simulink model "lab2_5_observer"  (R2023a)
settings: Solver=VariableStepAuto  StartTime=0.0  StopTime=2  RelTol=1e-3
values from neighbouring files (symbols this model uses):
  A = eye(3) + Ts * A    [part_deriv.m]
undefined symbols (not defined in the file or in its folder): B, C, K, L, u0, x10, x20, x30
settings Model: Creator=bz  LastModifiedBy=bz

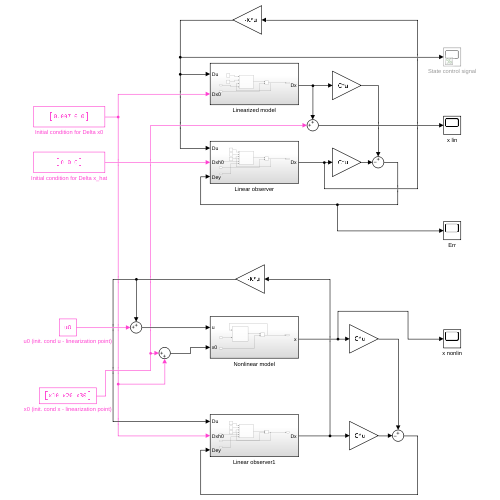
[thumbnail: Simulink's stored preview of the top-level diagram]
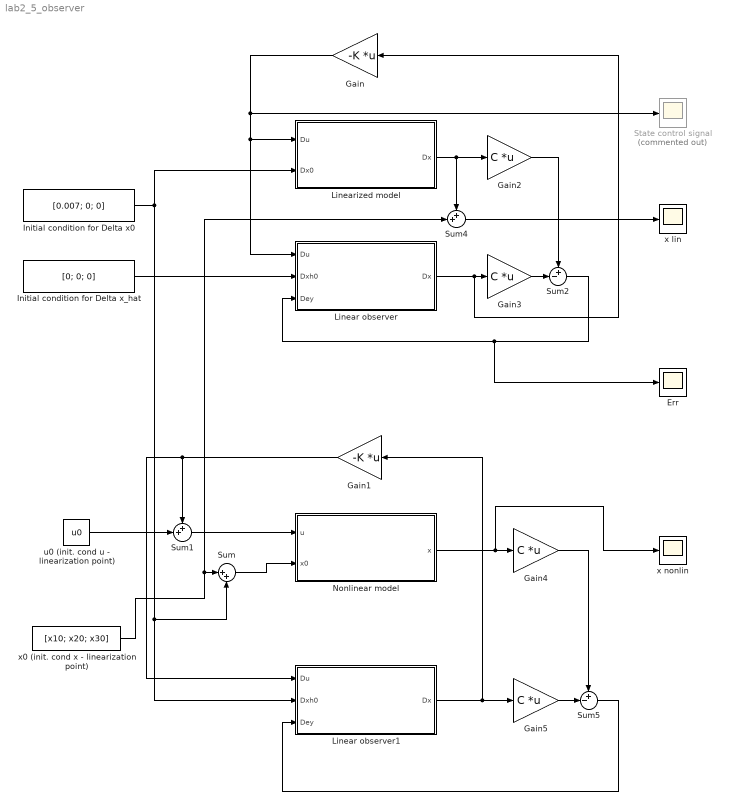
== system lab2_5_observer ==
  Err : Scope
  Gain : Gain  Gain=-K  Multiplication=Matrix(K*u)
  Gain1 : Gain  Gain=-K  Multiplication=Matrix(K*u)
  Gain{2..5} (4 alike) : Gain  Gain=C  Multiplication=Matrix(K*u)
  Initial condition for Delta x0 : Constant  Value=[0.007; 0; 0]
  Initial condition for Delta x_hat : Constant  Value=[0; 0; 0]
  Linear observer : Subsystem
  Linear observer1 : Subsystem
  Linearized model : Subsystem
  Nonlinear model : Subsystem
  State control signal : Scope  Commented=on
  Sum : Sum  Inputs=|++
  Sum1 : Sum  Inputs=++|
  Sum2 : Sum  Inputs=+-|
  Sum4 : Sum  Inputs=++|
  Sum5 : Sum  Inputs=+-|
  u0 (init. cond u - linearization point) : Constant  Value=u0
  x lin : Scope
  x nonlin : Scope
  x0 (init. cond x - linearization point) : Constant  Value=[x10; x20; x30]
  wires:
  Initial condition for Delta x0/1 -> Linear observer1/2(Dxh0), Sum/2, Linearized model/2(Dx0)
  x0 (init. cond x - linearization point)/1 -> Sum4/2, Sum/1
  Linearized model/1(Dx) -> Gain2/1, Sum4/1
  Sum1/1 -> Nonlinear model/1(u)
  Sum/1 -> Nonlinear model/2(x0)
  Nonlinear model/1(x) -> x nonlin/1, Gain4/1
  Gain/1 -> State control signal/1, Linearized model/1(Du), Linear observer/1(Du)
  Linear observer1/1(Dx) -> Gain5/1, Gain1/1
  Gain1/1 -> Linear observer1/1(Du), Sum1/1
  Gain2/1 -> Sum2/1
  Linear observer/1(Dx) -> Gain/1, Gain3/1
  Gain3/1 -> Sum2/2
  Sum2/1 -> Err/1, Linear observer/3(Dey)
  Sum4/1 -> x lin/1
  u0 (init. cond u - linearization point)/1 -> Sum1/2
  Gain4/1 -> Sum5/1
  Gain5/1 -> Sum5/2
  Sum5/1 -> Linear observer1/3(Dey)
  Initial condition for Delta x_hat/1 -> Linear observer/2(Dxh0)

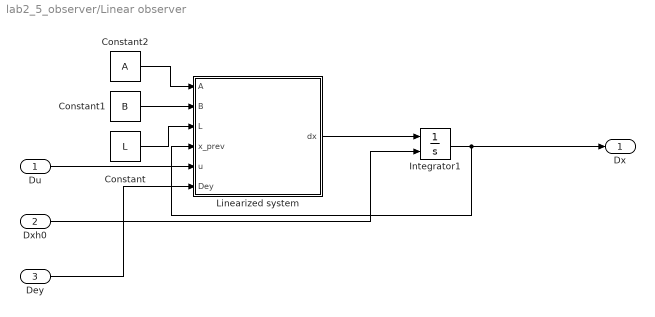
== system lab2_5_observer/Linear observer ==
  Du : Inport
  Dxh0 : Inport  Port=2
  Dey : Inport  Port=3
  Constant : Constant  Value=L
  Constant1 : Constant  Value=B
  Constant2 : Constant  Value=A
  Integrator1 : Integrator  InitialConditionSource=external
  Linearized system : MATLAB Function  TreatAsAtomicUnit=on
  Dx : Outport
  wires:
  Linearized system/1(dx) -> Integrator1/1
  Integrator1/1 -> Dx/1, Linearized system/4(x_prev)
  Dxh0/1 -> Integrator1/2
  Du/1 -> Linearized system/5(u)
  Dey/1 -> Linearized system/6(Dey)
  Constant/1 -> Linearized system/3(L)
  Constant1/1 -> Linearized system/2(B)
  Constant2/1 -> Linearized system/1(A)

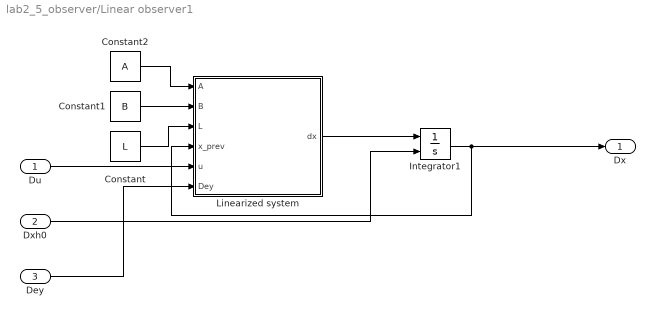
== system lab2_5_observer/Linear observer1 ==
  Du : Inport
  Dxh0 : Inport  Port=2
  Dey : Inport  Port=3
  Constant : Constant  Value=L
  Constant1 : Constant  Value=B
  Constant2 : Constant  Value=A
  Integrator1 : Integrator  InitialConditionSource=external
  Linearized system : MATLAB Function  TreatAsAtomicUnit=on
  Dx : Outport
  wires:
  Linearized system/1(dx) -> Integrator1/1
  Integrator1/1 -> Dx/1, Linearized system/4(x_prev)
  Dxh0/1 -> Integrator1/2
  Du/1 -> Linearized system/5(u)
  Dey/1 -> Linearized system/6(Dey)
  Constant/1 -> Linearized system/3(L)
  Constant1/1 -> Linearized system/2(B)
  Constant2/1 -> Linearized system/1(A)

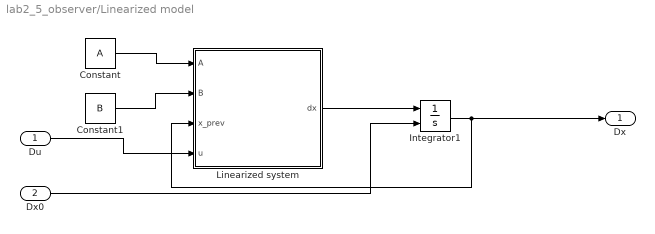
== system lab2_5_observer/Linearized model ==
  Du : Inport
  Dx0 : Inport  Port=2
  Constant : Constant  Value=A
  Constant1 : Constant  Value=B
  Integrator1 : Integrator  InitialConditionSource=external
  Linearized system : MATLAB Function  TreatAsAtomicUnit=on
  Dx : Outport
  wires:
  Linearized system/1(dx) -> Integrator1/1
  Integrator1/1 -> Dx/1, Linearized system/3(x_prev)
  Dx0/1 -> Integrator1/2
  Du/1 -> Linearized system/4(u)
  Constant/1 -> Linearized system/1(A)
  Constant1/1 -> Linearized system/2(B)

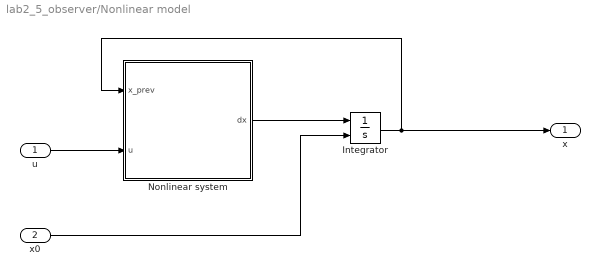
== system lab2_5_observer/Nonlinear model ==
  u : Inport
  x0 : Inport  Port=2
  Integrator : Integrator  InitialConditionSource=external
  Nonlinear system : MATLAB Function  TreatAsAtomicUnit=on
  x : Outport
  wires:
  Integrator/1 -> x/1, Nonlinear system/1(x_prev)
  Nonlinear system/1(dx) -> Integrator/1
  x0/1 -> Integrator/2
  u/1 -> Nonlinear system/2(u)

== matlab function lab2_5_observer/Linearized model/Linearized system ==
  data: A input; B input; x_prev input; u input; dx output size=[3,1]
function dx = fcn(A, B, x_prev, u)
% A = [0              0.0010      0;
%      1.6847         0           -0.0257;
%      0              0           -0.2888] * 1e3;
% 
% B = [0;
%      0;
%      1.2706] * 1e3;

dx = A * x_prev + B * u;

end

== matlab function lab2_5_observer/Nonlinear model/Nonlinear system ==
  data: x_prev input; u input; dx output size=[3,1]
function dx  = fcn(x_prev, u)

% x_prev
x1 = x_prev(1);
if x1 < 0
    x1 = 0;
end
x2 = x_prev(2);
x3 = x_prev(3);

FemP1 = 0.017521;
FemP2 = 0.0058231;

ci = -0.4;
ki = 4.4;
m = 0.016;
g = 9.81;

fiP1 = 1.4142e-4;
fiP2 = 4.5626e-3;

% fi = (fiP1/fiP2 * exp(-x1/fiP2));
% Fem1 = x3 ^ 2 * FemP1/FemP2 * exp(-x1/FemP2);

% x1_dot = 1;
% x2_dot = -Fem1/(2 * m) + g;
% x3_dot = 1/fi * (ki * u + ci - x3);

x1_dot = x2;
x2_dot = -(x3^2)*(FemP1/(FemP2*2*m))*exp(-x1/FemP2)+g;
x3_dot = 1/((fiP1/fiP2)*exp(-x1/fiP2))*(ki*u+ci-x3);

if x1_dot < 0
    x1_dot = 0;
end

% exp(-x1/FemP2)

dx = [x1_dot; x2_dot; x3_dot];

end

== matlab function lab2_5_observer/Linear observer/Linearized system ==
  data: A input; B input; L input; x_prev input; u input; dx output size=[3,1]; Dey input
function dx  = fcn(A, B, L, x_prev, u, Dey)

dx = A * x_prev + B * u + L * Dey;

end

== matlab function lab2_5_observer/Linear observer1/Linearized system ==
  data: A input; B input; L input; x_prev input; u input; dx output size=[3,1]; Dey input
function dx  = fcn(A, B, L, x_prev, u, Dey)

dx = A * x_prev + B * u + L * Dey;

end
